simulink model "wlan80211BeaconRx"  (R2014b)
settings: Solver=FixedStepDiscrete  SolverMode=SingleTasking  StartTime=0.0  StopTime=Inf  RelTol=1e-3
PreLoadFcn:
  | load('commwlan80211BusTypes')
  | openMPDUGUI = true;
  | sample = 860*2816;
PostLoadFcn:
  | wlan80211BeaconRxModelParams('init')
  | wlan80211BeaconRxModelParams('scope')
InitFcn:
  | load('commwlan80211BusTypes')
  | wlan80211BeaconRxModelParams('init')
model workspace: external: MAT-File (data not in the file)
values from neighbouring files (symbols this model uses):
  p80211 = commwlan80211BeaconRxInit(agcStepSize, agcMaxGain,        corrThreshold, sampsPerChip)    [sdruwlan80211BeaconRxInit.m]    (also in sdruwlan80211BeaconRxModelParams.m = sdruwlan80211BeaconRxInit(agcStepSize, agcMaxGain,        co; wlan80211BeaconRxModelParams.m = wlan80211BeaconRxInit(agcStepSize, agcMaxGain,              )
libraries: commwlan80211BeaconLib x7, commdigbbndpm3 x1, dspsigops x1, commsequence2 x1, commfilt2 x1, simulink x1
CloseFcn:
  | clear sample BeaconFrameBodyType BeaconMPDUType CapabilityType FrameCtrlType InfoElementType MPDUHeaderType p80211 commwlan80211TxFilt rcvd openMPDUGUI mpduFigPos
  | hFig = findall(0, 'Type', 'figure', 'Name', '802.11 Beacon Frame');
  | if ishghandle(hFig)
  | close(hFig);
  | end
  | clear hFig
  | if (exist('ans')==1) && (iscell(ans) && (numel(ans) == 0))
  | clear ans
  | end
Description:
  | IEEE 802.11 WLAN Beacon Frame Receiver for USRP(R)
  | 
  | This example shows how to process a beacon frame captured with USRP and display the
  | frame information.
settings Model: Creator=The MathWorks Inc.  LastModifiedBy=DPu1
settings DataIOCC: SaveOutput=off  SignalLogging=off  DSMLogging=off  SaveTime=off
settings OptimizationCC: InlineParams=on  InlineInvariantSignals=on  ExpressionDepthLimit=2147483647  EfficientFloat2IntCast=on
settings DebuggingCC: UnderspecifiedInitializationDetection=Classic  MergeDetectMultiDrivingBlocksExec=none  UniqueDataStoreMsg=error  StateNameClashWarn=warning
settings RTWCC: CustomSourceCode=|
  | #include <stdio.h>
  | #include <stdlib.h>
settings GRTTargetCC: CombineOutputUpdateFcns=off  GRTInterface=on

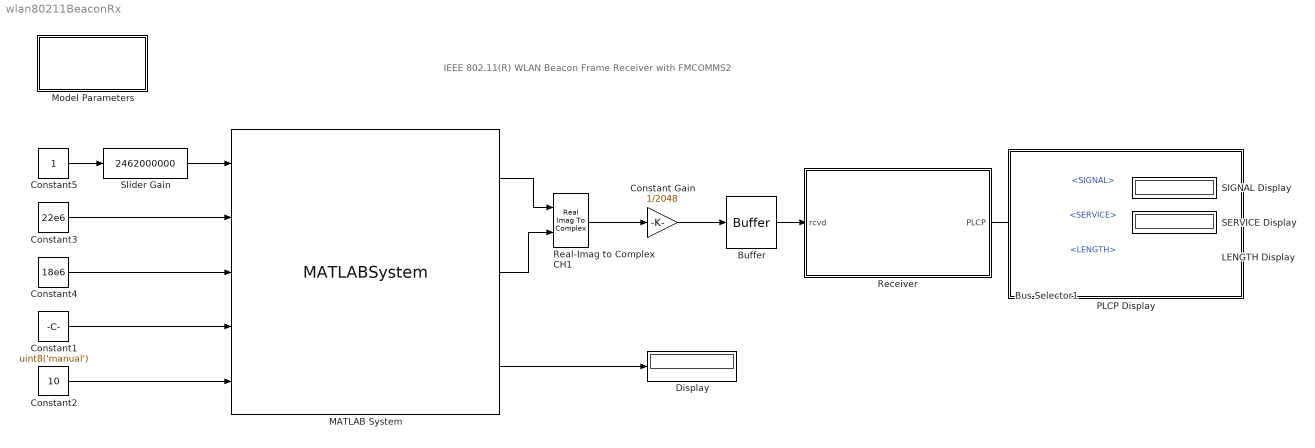
== system wlan80211BeaconRx ==
  note: IEEE 802.11(R) WLAN
      | Beacon Frame Receiver with FMCOMMS2
  Buffer : Buffer  N=2816  TreatMby1Signals=One channel
  Bus Selector1 : BusSelector  OutputSignals=SIGNAL,SERVICE,LENGTH
  Constant Gain : Gain  Gain=1/2048  SaturateOnIntegerOverflow=on  ParamDataTypeStr=Inherit: Same as input
  Constant1 : Constant  Value=uint8('manual')  SampleTime=1
  Constant2 : Constant  Value=10  SampleTime=1
  Constant3 : Constant  Value=22e6  SampleTime=1
  Constant4 : Constant  Value=18e6  SampleTime=1
  Constant5 : Constant  SampleTime=1
  Display : Display
  LENGTH Display : Display
  MATLAB System : MATLABSystem  System=iio_sys_obj  SimulateUsing=Interpreted execution  ip_address=10.66.99.142  dev_name=ad9361  in_ch_no=0  in_ch_size=sample  out_ch_no=2  out_ch_size=sample
      mask Type: iio_sys_obj
      mask Display:
      | disp('ad9361');
      | port_label('input',1,'RX_LO_FREQ');
      | port_label('input',2,'RX_SAMPLING_FREQ');
      | port_label('input',3,'RX_RF_BANDWIDTH');
      | port_label('input',4,'RX1_GAIN_MODE');
      | port_label('input',5,'RX1_GAIN');
      | port_label('output',1,'DATA_OUT1');
      | port_label('output',2,'DATA_OUT2');
      | port_label('output',3,'RX1_RSSI');
  Model Parameters : Subsystem  mask(Model Parameters){chanNum=11, agcStepSize=5e-3, agcMaxGain=27, corrThreshold=15e3}
      mask prompts: chanNum "Channel number"; agcStepSize "AGC step size:"; agcMaxGain "Maximum AGC gain:"; corrThreshold "Synchronization threshold:"
      mask help:
      | Choose 802.11 receiver parameters.
      |
      | You can select channel number for the 802.11 signals. You can set the AGC parameters and samples per chip used in the receiver. You can also set the synchronization threshold value to determine the correlation threshold used to declare the presence of an 802.11 packet.
      mask init:
      | wlan80211BeaconRxModelParams('init');
      mask Help: web(usrpdhelp, '-helpbrowser');
      mask TypeOptions chanNum: 1 | 2 | 3 | 4 | 5 | 6 | 7 | 8 | 9 | 10 | 11
      mask Display: disp('Model\nParameters')
  PLCP Display : Subsystem
      mask Display: disp('')
  Real-Imag to Complex CH1 : RealImagToComplex  SampleTime=sample/(25e6)
  Receiver : Subsystem
  SERVICE Display : Display
      settings: Format=hex (Stored Integer)
  SIGNAL Display : Display
      settings: Format=hex (Stored Integer)
  Slider Gain : simulink/Math Operations/Slider Gain  low=200000  gain=2462000000  high=6000000000
  wires:
  Bus Selector1/3 -> LENGTH Display/1  "<LENGTH>"
  Bus Selector1/1 -> SIGNAL Display/1  "<SIGNAL>"
  Bus Selector1/2 -> SERVICE Display/1  "<SERVICE>"
  Receiver/1(PLCP) -> Bus Selector1/1
  Real-Imag to Complex CH1/1 -> Constant Gain/1
  Constant Gain/1 -> Buffer/1
  Buffer/1 -> Receiver/1(rcvd)
  Constant5/1 -> Slider Gain/1
  Slider Gain/1 -> MATLAB System/1
  Constant3/1 -> MATLAB System/2
  Constant4/1 -> MATLAB System/3
  Constant1/1 -> MATLAB System/4
  Constant2/1 -> MATLAB System/5
  MATLAB System/3 -> Display/1
  MATLAB System/1 -> Real-Imag to Complex CH1/1
  MATLAB System/2 -> Real-Imag to Complex CH1/2

== system wlan80211BeaconRx/Model Parameters ==

== system wlan80211BeaconRx/PLCP Display ==

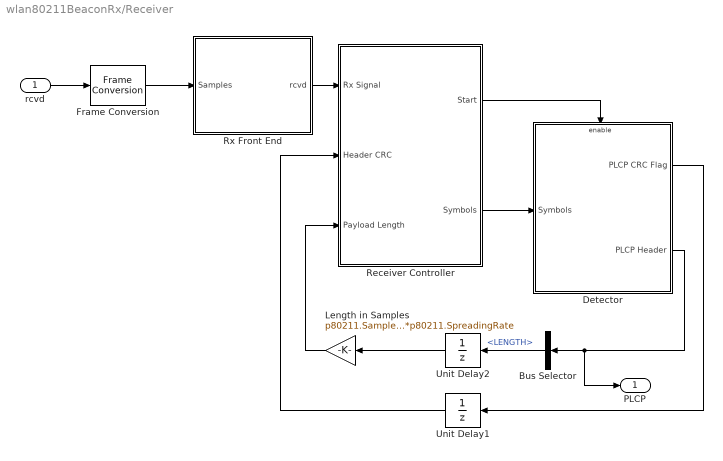
== system wlan80211BeaconRx/Receiver ==
  rcvd : Inport
  Bus Selector : BusSelector  OutputSignals=LENGTH
  Detector : Subsystem
      settings: CloseFcn=clear BeaconFrameBodyType rcvd
  Frame Conversion : FrameConversion
  Length in Samples : Gain  Gain=p80211.SamplesPerChip*p80211.SpreadingRate  OutDataTypeStr=uint32  SaturateOnIntegerOverflow=on  ParamDataTypeStr=Inherit: Same as input
  Receiver Controller : Subsystem
  Rx Front End : Subsystem
  Unit Delay1 : UnitDelay  InitialCondition=1  SampleTime=-1
  Unit Delay2 : UnitDelay  InitialCondition=1  SampleTime=-1
  PLCP : Outport
  wires:
  Receiver Controller/2(Symbols) -> Detector/1(Symbols)
  Detector/2(PLCP Header) -> PLCP/1, Bus Selector/1
  Length in Samples/1 -> Receiver Controller/3(Payload Length)
  Unit Delay2/1 -> Length in Samples/1
  Bus Selector/1 -> Unit Delay2/1  "<LENGTH>"
  Unit Delay1/1 -> Receiver Controller/2(Header CRC)
  Rx Front End/1(rcvd) -> Receiver Controller/1(Rx Signal)
  Detector/1(PLCP CRC Flag) -> Unit Delay1/1
  Receiver Controller/1(Start) -> Detector/Enable
  rcvd/1 -> Frame Conversion/1
  Frame Conversion/1 -> Rx Front End/1(Samples)

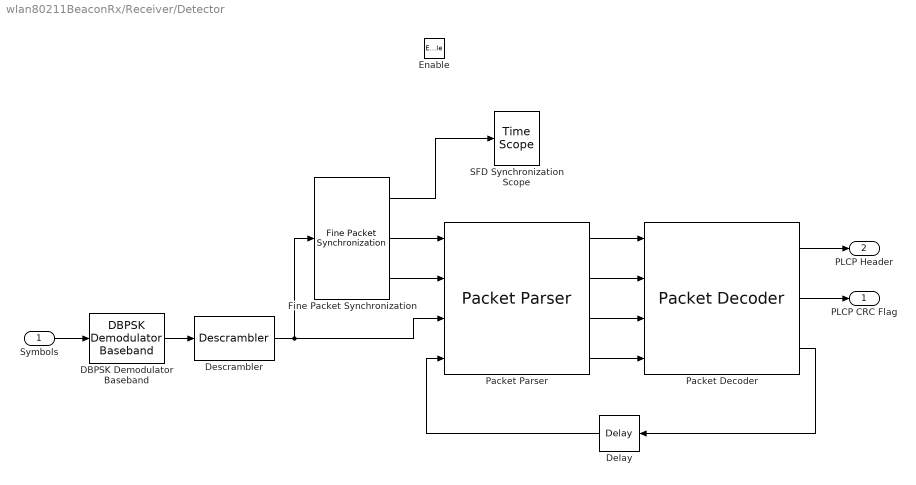
== system wlan80211BeaconRx/Receiver/Detector ==
  Symbols : Inport
  Enable : EnablePort  StatesWhenEnabling=reset  PropagateVarSize=During execution
  DBPSK Demodulator Baseband : commdigbbndpm3/DBPSK Demodulator Baseband  Ph=0  outDtype=Smallest unsigned integer
  Delay : dspsigops/Delay  InputProcessing=Columns as channels (frame based)  dly_unit=Samples  delay=1  ic_detail=off  dif_ic_for_ch=off  dif_ic_for_dly=off  ic=0  reset_popup=None
  Descrambler : commsequence2/Descrambler  M=2  poly=p80211.ScramblerPolynomial  iniStaSource=Dialog Parameter  ini_sta=[0 0 0 0 0 0 0]  resetViaPort=off
  Fine Packet Synchronization : commwlan80211BeaconLib/Fine Packet Synchronization
  Packet Decoder : commwlan80211BeaconLib/Packet Decoder
  Packet Parser : commwlan80211BeaconLib/Packet Parser
  SFD Synchronization Scope : TimeScope  Priority=10  DefaultConfigurationName=spbscopes.TimeScopeBlockCfg
  PLCP CRC Flag : Outport  InitialOutput=1
  PLCP Header : Outport  Port=2
  wires:
  Packet Decoder/3 -> Delay/1
  Packet Decoder/2 -> PLCP CRC Flag/1
  Packet Decoder/1 -> PLCP Header/1
  Packet Parser/4 -> Packet Decoder/4
  Packet Parser/3 -> Packet Decoder/3
  Packet Parser/2 -> Packet Decoder/2
  Packet Parser/1 -> Packet Decoder/1
  Delay/1 -> Packet Parser/4
  Fine Packet Synchronization/3 -> Packet Parser/2
  Fine Packet Synchronization/2 -> Packet Parser/1
  Descrambler/1 -> Packet Parser/3, Fine Packet Synchronization/1
  Symbols/1 -> DBPSK Demodulator Baseband/1
  DBPSK Demodulator Baseband/1 -> Descrambler/1
  Fine Packet Synchronization/1 -> SFD Synchronization Scope/1

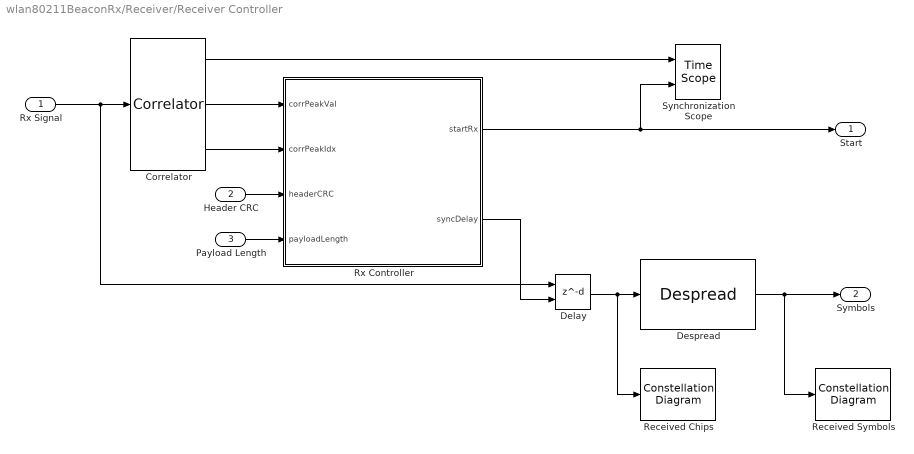
== system wlan80211BeaconRx/Receiver/Receiver Controller ==
  Rx Signal : Inport
  Header CRC : Inport  Port=2
  Payload Length : Inport  Port=3
  Correlator : commwlan80211BeaconLib/Correlator
  Delay : Delay  DelayLengthSource=Input port  DelayLengthUpperLimit=p80211.SamplesPerChannelFrame  InputProcessing=Columns as channels (frame based)
      settings: InputPortMap=u0,p1
  Despread : commwlan80211BeaconLib/Despread
  Received Chips : ConstellationDiagram  Tag=ScatterPlot  Priority=1
  Received Symbols : ConstellationDiagram  Tag=ScatterPlot  Priority=2
  Rx Controller : MATLAB Function  TreatAsAtomicUnit=on
  Synchronization Scope : TimeScope  Priority=1  DefaultConfigurationName=spbscopes.TimeScopeBlockCfg  NumInputPorts=2
  Start : Outport
  Symbols : Outport  Port=2
  wires:
  Despread/1 -> Received Symbols/1, Symbols/1
  Rx Controller/2(syncDelay) -> Delay/2
  Rx Controller/1(startRx) -> Synchronization Scope/2, Start/1
  Header CRC/1 -> Rx Controller/3(headerCRC)
  Correlator/2 -> Rx Controller/1(corrPeakVal)
  Correlator/3 -> Rx Controller/2(corrPeakIdx)
  Rx Signal/1 -> Correlator/1, Delay/1
  Payload Length/1 -> Rx Controller/4(payloadLength)
  Delay/1 -> Despread/1, Received Chips/1
  Correlator/1 -> Synchronization Scope/1

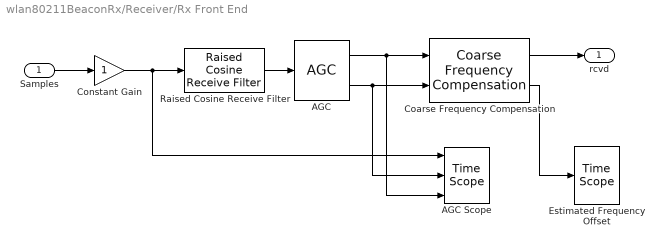
== system wlan80211BeaconRx/Receiver/Rx Front End ==
  Samples : Inport
  AGC : commwlan80211BeaconLib/AGC
  AGC Scope : TimeScope  DefaultConfigurationName=spbscopes.TimeScopeBlockCfg  NumInputPorts=3
  Coarse Frequency Compensation : commwlan80211BeaconLib/Coarse Frequency Compensation  decimRate=44  maxOffset=50000  M=2
  Constant Gain : Gain  SaturateOnIntegerOverflow=on  ParamDataTypeStr=Inherit: Same as input
  Estimated Frequency Offset : TimeScope  DefaultConfigurationName=spbscopes.TimeScopeBlockCfg
  Raised Cosine Receive Filter : commfilt2/Raised Cosine Receive Filter  filtType=Square root  N=p80211.SamplesPerChip  filtSpan=p80211.FilterOrder  currentFiltSpan=p80211.FilterOrder  D=(p80211.FilterOrder)/2  R=0.3  sampMode=Mute  saveAsFlag=0  rateMode=Downsampling  downFactor=1  downOffset=0  framing=Enforce single-rate processing  InputProcessing=Columns as channels (frame based)  checkGain=Normalized  filterGain=1  checkCoeff=off  variableName=rcRxFilt  launchFVT=off  roundingMode=Floor  overflowMode=off
  rcvd : Outport
  wires:
  Coarse Frequency Compensation/1 -> rcvd/1
  AGC/1 -> Coarse Frequency Compensation/1, AGC Scope/3
  Raised Cosine Receive Filter/1 -> AGC/1
  Coarse Frequency Compensation/2 -> Estimated Frequency Offset/1
  AGC/2 -> AGC Scope/2, Coarse Frequency Compensation/2
  Samples/1 -> Constant Gain/1
  Constant Gain/1 -> Raised Cosine Receive Filter/1, AGC Scope/1

== matlab function wlan80211BeaconRx/Receiver/Receiver Controller/Rx Controller ==
  data: corrPeakVal input; startRx output; corrPeakIdx input; headerCRC input boolean size=[1 1]; payloadLength input size=1; p80211 parameter; syncDelay output
function [startRx, syncDelay] = ...
  rxCtrl(corrPeakVal, corrPeakIdx, headerCRC, payloadLength, p80211)
%#codegen

persistent rxOn controllerState payloadCount lastSyncDelay corrPeakValOld

% State Enums
SearchPLCP = 0;
GetPLCP    = 2;
GetPayload = 4;

if isempty(rxOn)
  % Initialize receiver controller
  rxOn = false;
  controllerState = SearchPLCP;
  payloadCount = 0;
  lastSyncDelay = 0;
  corrPeakValOld = 0;
end

if (corrPeakValOld < corrPeakVal)
  controllerState = SearchPLCP;
end

switch controllerState
  case SearchPLCP
    % Search for the PLCP SYNC signal
    
    if corrPeakVal > p80211.CorrelationThreshold
      corrPeakValOld = corrPeakVal;
      % Synchronize to the end of the SYNC. Get 8 (scrambler length) extra
      % bits to initialize DPSK demodulator and scrambler
      scramblerLen = length(p80211.ScramblerPolynomial);
      lastSyncDelay = p80211.SamplesPerChannelFrame - (corrPeakIdx ...
        - scramblerLen*p80211.SpreadingRate*p80211.SamplesPerChip); 
      payloadCount = p80211.NumSYNCSamples ...
        - scramblerLen*p80211.SpreadingRate*p80211.SamplesPerChip;
      rxOn = true;
      
      controllerState = GetPLCP;
    end
  case GetPLCP
    % In this state we receive both SFD, which is part of PLCP preamble,
    % and the PLCP header
    
    payloadCount = payloadCount + p80211.SamplesPerChannelFrame;
    
    if (payloadCount >= ...
        (p80211.NumPLCPSamples+p80211.ScramblerAmbiguitySamples))
      if headerCRC ~= 1
        controllerState = GetPayload;
      else
        rxOn = false;
        lastSyncDelay = 0;
        payloadCount = 0;
        controllerState = SearchPLCP;
      end
    end
  case GetPayload
    % Receive payload symbols
    
    payloadCount = payloadCount + p80211.SamplesPerChannelFrame;
    
    if payloadCount >= ...
        ((p80211.NumPLCPSamples+p80211.ScramblerAmbiguitySamples) + ...
        payloadLength)
      rxOn = false;
      lastSyncDelay = 0;
      payloadCount = 0;
      controllerState = SearchPLCP;
    end
end

startRx = rxOn;
syncDelay = lastSyncDelay;
